simulink model "BLDC_ClosedLoop_s32k144"  (Simulink 9.0)
settings: Solver=FixedStepDiscrete  StartTime=0.0  StopTime=10.0  FixedStep=0.1  RelTol=1e-3  EnableMultiTasking=on
InitFcn:
  | mbd_s32k_consistency_checks(bdroot(gcs));
undefined symbols (not defined in the file): External, LQFP, One, Shot, TRGMUX_PDB_TRIG
libraries: mbd_s32k1xx_ec_toolbox x45, simulink x10, mbd_msd_ec_toolbox x5, ammclib_bam_s32k14x x2
(part 2 of 2)

== system BLDC_ClosedLoop_s32k144/S32K144 EVB/10us_interrupt/MeasureHallSignal_HighEdge_Time/reset counter ==
  Action Port : ActionPort  ActionPortLabel=else
  Data Store Write : DataStoreWrite  DataStoreName=SPD_COUNTS
  zero : Constant  Value=0  OutDataTypeStr=uint32
  wires:
  zero/1 -> Data Store Write/1

== system BLDC_ClosedLoop_s32k144/S32K144 EVB/Control_Logic/enable_FTM_PDB_ADC_triggering/Custom code to reload the PDB value ==

== system BLDC_ClosedLoop_s32k144/S32K144 EVB/Event_Control/ControlEventLogic/Function-Call Subsystem ==
  function : TriggerPort  TriggerType=function-call  VariantControl=Variant
  Add : Sum  AccumDataTypeStr=uint32
  Constant : Constant  OutDataTypeStr=uint32
  Data Store Read : DataStoreRead  DataStoreName=HallChangeCount  DataStoreElements=HallChangeCount
  Data Store Write : DataStoreWrite  DataStoreName=HallChangeCount  DataStoreElements=HallChangeCount
  Function-Call Generator : simulink/Ports & Subsystems/Function-Call Generator  sample_time=-1  numberOfIterations=1
  Call : Outport
  wires:
  Function-Call Generator/1 -> Call/1
  Data Store Read/1 -> Add/1
  Constant/1 -> Add/2
  Add/1 -> Data Store Write/1

== system BLDC_ClosedLoop_s32k144/S32K144 EVB/Event_Control/ControlEventLogic/Toggle_HallA ==
  function : TriggerPort  TriggerType=function-call  VariantControl=Variant
  Data Store Read1 : DataStoreRead  DataStoreName=Hall_A_sensor
  Data Store Write1 : DataStoreWrite  DataStoreName=Hall_A_sensor
  Function-Call Generator : simulink/Ports & Subsystems/Function-Call Generator  sample_time=-1  numberOfIterations=1
  Logical Operator : Logic  Operator=NOT  AllPortsSameDT=off  OutDataTypeStr=boolean
  Call : Outport
  wires:
  Function-Call Generator/1 -> Call/1
  Data Store Read1/1 -> Logical Operator/1
  Logical Operator/1 -> Data Store Write1/1

== system BLDC_ClosedLoop_s32k144/S32K144 EVB/Event_Control/ControlEventLogic/Toggle_HallB ==
  function : TriggerPort  TriggerType=function-call  VariantControl=Variant
  Data Store Read1 : DataStoreRead  DataStoreName=Hall_B_sensor
  Data Store Write1 : DataStoreWrite  DataStoreName=Hall_B_sensor
  Function-Call Generator : simulink/Ports & Subsystems/Function-Call Generator  sample_time=-1  numberOfIterations=1
  Logical Operator : Logic  Operator=NOT  AllPortsSameDT=off  OutDataTypeStr=boolean
  Call : Outport
  wires:
  Function-Call Generator/1 -> Call/1
  Data Store Read1/1 -> Logical Operator/1
  Logical Operator/1 -> Data Store Write1/1

== system BLDC_ClosedLoop_s32k144/S32K144 EVB/Event_Control/ControlEventLogic/Toggle_HallC ==
  function : TriggerPort  TriggerType=function-call  VariantControl=Variant
  Data Store Read1 : DataStoreRead  DataStoreName=Hall_C_sensor
  Data Store Write1 : DataStoreWrite  DataStoreName=Hall_C_sensor
  Function-Call Generator : simulink/Ports & Subsystems/Function-Call Generator  sample_time=-1  numberOfIterations=1
  Logical Operator : Logic  Operator=NOT  AllPortsSameDT=off  OutDataTypeStr=boolean
  Call : Outport
  wires:
  Function-Call Generator/1 -> Call/1
  Data Store Read1/1 -> Logical Operator/1
  Logical Operator/1 -> Data Store Write1/1

== system BLDC_ClosedLoop_s32k144/S32K144 EVB/Hall_Emulation_Sequence/Speed Estimator/keep updating history ==
  Action Port : ActionPort  ActionPortLabel=else
  Data Store Read : DataStoreRead  DataStoreName=Hall_A_sensor
  Data Store Write3 : DataStoreWrite  DataStoreName=HALL_A_Input_1
  wires:
  Data Store Read/1 -> Data Store Write3/1

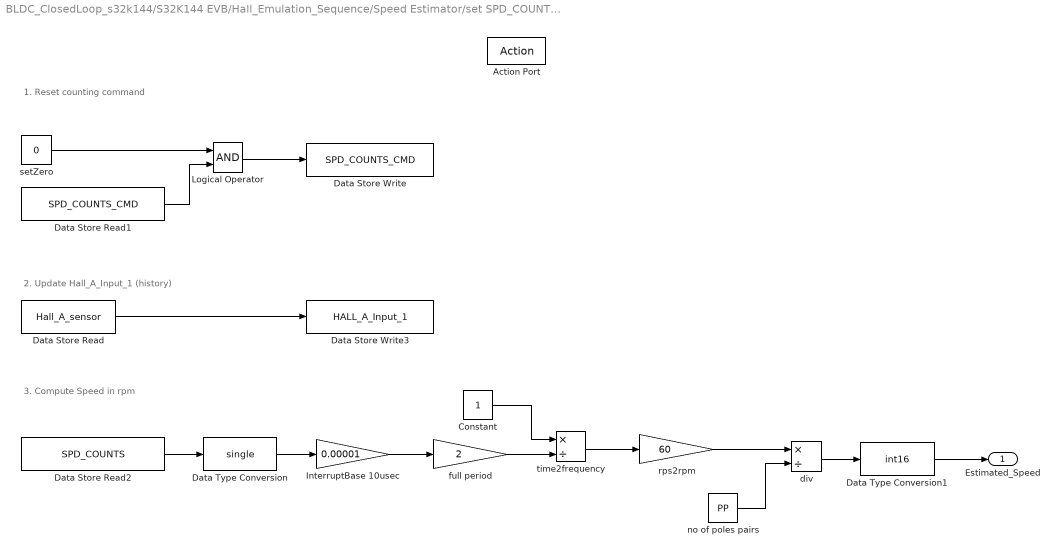
== system BLDC_ClosedLoop_s32k144/S32K144 EVB/Hall_Emulation_Sequence/Speed Estimator/set SPD_COUNT_CMD = 0 ==
  note: 2. Update Hall_A_Input_1 (history)
  note: 1. Reset counting command
  note: 3. Compute Speed in rpm
  Action Port : ActionPort  ActionPortLabel=elseif((u1 == 0)&(u2 == 1))
  Constant : Constant  OutDataTypeStr=single
  Data Store Read : DataStoreRead  DataStoreName=Hall_A_sensor
  Data Store Read1 : DataStoreRead  DataStoreName=SPD_COUNTS_CMD
  Data Store Read2 : DataStoreRead  DataStoreName=SPD_COUNTS
  Data Store Write : DataStoreWrite  DataStoreName=SPD_COUNTS_CMD
  Data Store Write3 : DataStoreWrite  DataStoreName=HALL_A_Input_1
  Data Type Conversion : DataTypeConversion  OutDataTypeStr=single
  Data Type Conversion1 : DataTypeConversion  OutDataTypeStr=int16
  InterruptBase 10usec : Gain  Gain=0.00001  OutDataTypeStr=single
  Logical Operator : Logic  AllPortsSameDT=off  OutDataTypeStr=boolean
  div : Product  Inputs=*/  OutDataTypeStr=single
  full period : Gain  Gain=2  OutDataTypeStr=single
  no of poles pairs : Constant  Value=PP  OutDataTypeStr=single
  rps2rpm : Gain  Gain=60  OutDataTypeStr=single
  setZero : Constant  Value=0  OutDataTypeStr=boolean
  time2frequency : Product  Inputs=*/  OutDataTypeStr=single
  Estimated_Speed : Outport
  wires:
  Data Store Read/1 -> Data Store Write3/1
  Logical Operator/1 -> Data Store Write/1
  setZero/1 -> Logical Operator/1
  Data Store Read1/1 -> Logical Operator/2
  Data Store Read2/1 -> Data Type Conversion/1
  Data Type Conversion/1 -> InterruptBase 10usec/1
  InterruptBase 10usec/1 -> full period/1
  full period/1 -> time2frequency/2
  Constant/1 -> time2frequency/1
  time2frequency/1 -> rps2rpm/1
  rps2rpm/1 -> div/1
  no of poles pairs/1 -> div/2
  div/1 -> Data Type Conversion1/1
  Data Type Conversion1/1 -> Estimated_Speed/1

== system BLDC_ClosedLoop_s32k144/S32K144 EVB/Hall_Emulation_Sequence/Speed Estimator/set SPD_COUNT_CMD = 1 ==
  note: 2. Update Hall_A_Input_1 (history)
  note: 1. Enable counting command
  Action Port : ActionPort  ActionPortLabel=if((u1 == 1)&(u2 == 0))
  Data Store Read : DataStoreRead  DataStoreName=Hall_A_sensor
  Data Store Read1 : DataStoreRead  DataStoreName=SPD_COUNTS_CMD
  Data Store Write : DataStoreWrite  DataStoreName=SPD_COUNTS_CMD
  Data Store Write3 : DataStoreWrite  DataStoreName=HALL_A_Input_1
  Logical Operator : Logic  Operator=OR  AllPortsSameDT=off  OutDataTypeStr=boolean
  setOne : Constant  OutDataTypeStr=boolean
  wires:
  Data Store Read/1 -> Data Store Write3/1
  Logical Operator/1 -> Data Store Write/1
  setOne/1 -> Logical Operator/1
  Data Store Read1/1 -> Logical Operator/2

== system BLDC_ClosedLoop_s32k144/S32K144 EVB/IO Controls /Subsystem/Fault ==
  Action Port : ActionPort  ActionPortLabel=elseif((u2 == 1))
  BLUE : mbd_s32k1xx_ec_toolbox/GPIO Blocks/Digital_Output  gpio_pin=PTD0: [PTD0 | Port D I/O]  init_val=Low  drive_strength=Low
  GREEN : mbd_s32k1xx_ec_toolbox/GPIO Blocks/Digital_Output  gpio_pin=PTD16: [PTD16 | Port D I/O]  init_val=Low  drive_strength=Low
  OFF : Constant  OutDataTypeStr=boolean
  "OFF " : Constant  OutDataTypeStr=boolean
  "OFF  " : Constant  Value=0  OutDataTypeStr=boolean
  "ON " : Constant  Value=0  OutDataTypeStr=boolean
  RED : mbd_s32k1xx_ec_toolbox/GPIO Blocks/Digital_Output  gpio_pin=PTD15: [PTD15 | Port D I/O]  init_val=Low  drive_strength=Low
  "SpeedCmd " : DataStoreWrite  DataStoreName=START
  SpeedCmd 1 : DataStoreWrite  DataStoreName=READY
  wires:
  "OFF "/1 -> GREEN/1
  "ON "/1 -> RED/1
  OFF/1 -> BLUE/1
  "OFF  "/1 -> "SpeedCmd "/1, SpeedCmd 1/1

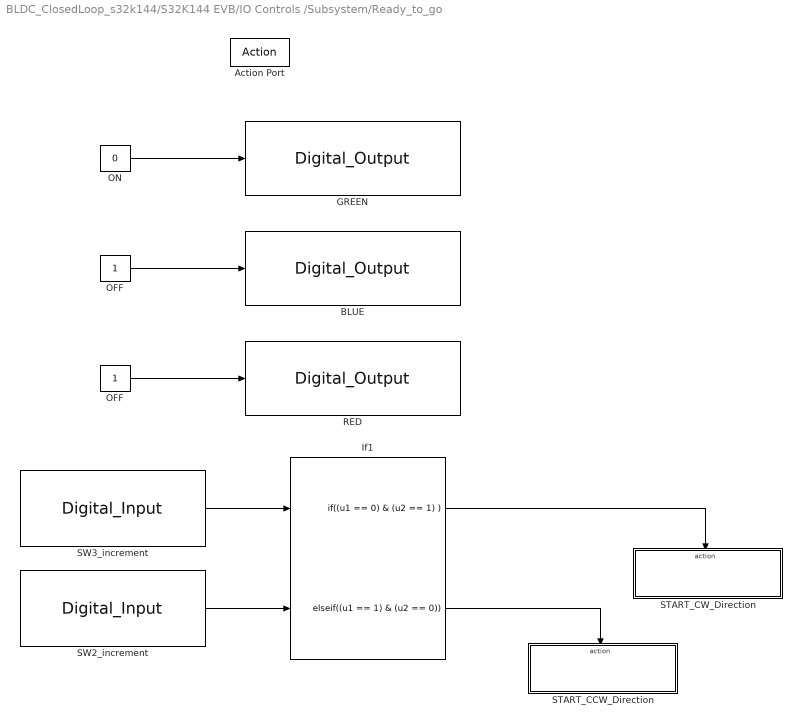
== system BLDC_ClosedLoop_s32k144/S32K144 EVB/IO Controls /Subsystem/Ready_to_go ==
  Action Port : ActionPort  ActionPortLabel=if((u1 == 0) & (u2 == 0))
  BLUE : mbd_s32k1xx_ec_toolbox/GPIO Blocks/Digital_Output  gpio_pin=PTD0: [PTD0 | Port D I/O]  init_val=Low  drive_strength=Low
  GREEN : mbd_s32k1xx_ec_toolbox/GPIO Blocks/Digital_Output  gpio_pin=PTD16: [PTD16 | Port D I/O]  init_val=Low  drive_strength=Low
  If1 : If  NumInputs=2  IfExpression=(u1 == 0) & (u2 == 1)  ElseIfExpressions=(u1 == 1) & (u2 == 0)  ShowElse=off
  "OFF " : Constant  OutDataTypeStr=boolean
  "OFF  " : Constant  OutDataTypeStr=boolean
  "ON  " : Constant  Value=0  OutDataTypeStr=boolean
  RED : mbd_s32k1xx_ec_toolbox/GPIO Blocks/Digital_Output  gpio_pin=PTD15: [PTD15 | Port D I/O]  init_val=Low  drive_strength=Low
  START_CCW_Direction : Subsystem  TreatAsAtomicUnit=on
  START_CW_Direction : Subsystem  TreatAsAtomicUnit=on
  SW2_increment : mbd_s32k1xx_ec_toolbox/GPIO Blocks/Digital_Input  gpio_pin=PTC12: [PTC12 | Port C I/O]  pull_resistor=None  passive_filter=off
  SW3_increment : mbd_s32k1xx_ec_toolbox/GPIO Blocks/Digital_Input  gpio_pin=PTC13: [PTC13 | Port C I/O]  pull_resistor=None  passive_filter=off
  wires:
  "ON  "/1 -> GREEN/1
  "OFF "/1 -> RED/1
  "OFF  "/1 -> BLUE/1
  If1/1 -> START_CW_Direction/Action
  SW3_increment/1 -> If1/1
  SW2_increment/1 -> If1/2
  If1/2 -> START_CCW_Direction/Action

== system BLDC_ClosedLoop_s32k144/S32K144 EVB/IO Controls /Subsystem/Running ==
  Action Port : ActionPort  ActionPortLabel=else
  BLUE : mbd_s32k1xx_ec_toolbox/GPIO Blocks/Digital_Output  gpio_pin=PTD0: [PTD0 | Port D I/O]  init_val=Low  drive_strength=Low
  GREEN : mbd_s32k1xx_ec_toolbox/GPIO Blocks/Digital_Output  gpio_pin=PTD16: [PTD16 | Port D I/O]  init_val=Low  drive_strength=Low
  "OFF " : Constant  OutDataTypeStr=boolean
  OFF_RED : Constant  OutDataTypeStr=boolean
  "ON " : Constant  Value=0  OutDataTypeStr=boolean
  RED : mbd_s32k1xx_ec_toolbox/GPIO Blocks/Digital_Output  gpio_pin=PTD15: [PTD15 | Port D I/O]  init_val=Low  drive_strength=Low
  wires:
  "OFF "/1 -> GREEN/1
  OFF_RED/1 -> RED/1
  "ON "/1 -> BLUE/1

== system BLDC_ClosedLoop_s32k144/S32K144 EVB/Protection_Check/Subsystem/FAILURE ==
  Action Port : ActionPort  ActionPortLabel=if((u1 < VDC_UNDERVOLTAGE) | (u1 > VDC_OVERVOLTAGE) | (u2 > IDC_OVERCURRENT))
  FAULT_write : DataStoreWrite  DataStoreName=FAULT
  FTM_PWM_Disable_Enable : mbd_s32k1xx_ec_toolbox/Motor Control Blocks/FTM Blocks/FTM_PWM_Disable_Enable  ftmModule=3  action=Disable
  NOK : Constant  OutDataTypeStr=boolean
  TPP_Functional_Mode : mbd_msd_ec_toolbox/TPP/TPP_Functional_Mode  tppInstance=0  action=Sleep
  wires:
  NOK/1 -> FAULT_write/1

== system BLDC_ClosedLoop_s32k144/S32K144 EVB/Trapezoidal_Control/SixStepCommutationLogic/Alignment_Counter ==
  Action Port : ActionPort  ActionPortLabel=if((u1 == 1))
  Align Sequence : Stateflow chart  TreatAsAtomicUnit=on
  AlignTimerIn : DataStoreRead  DataStoreName=AlignTimer
  AlignTimerOut : DataStoreWrite  DataStoreName=AlignTimer
  ExecureAlign : DataStoreWrite  DataStoreName=ExecuteAlign
  wires:
  Align Sequence/2(ExecuteAlign) -> ExecureAlign/1
  Align Sequence/1(DelayTimeOut) -> AlignTimerOut/1
  AlignTimerIn/1 -> Align Sequence/1(DelayTimeIn)

== system BLDC_ClosedLoop_s32k144/S32K144 EVB/Trapezoidal_Control/SixStepCommutationLogic/Do_Alignment ==
  DIR : Inport
  Action Port : ActionPort  ActionPortLabel=if((u1 == 1) & (u2 == 0) & (u3 == 1))
  CCW Dir : Subsystem
  CW Dir : Subsystem
  DirectionChk : If  Priority=1  IfExpression=(u1 >= 0)
  Merge : Merge
  Merge1 : Merge
  Merge2 : Merge
  Phase_A : Outport
  Phase_B : Outport  Port=2
  Phase_C : Outport  Port=3
  wires:
  DIR/1 -> DirectionChk/1
  DirectionChk/1 -> CW Dir/Action
  DirectionChk/2 -> CCW Dir/Action
  Merge/1 -> Phase_A/1
  Merge1/1 -> Phase_C/1
  CCW Dir/3(Out3) -> Merge1/2
  CW Dir/3(Out3) -> Merge1/1
  CW Dir/1(Out1) -> Merge/1
  CCW Dir/1(Out1) -> Merge/2
  CW Dir/2(Out2) -> Merge2/1
  CCW Dir/2(Out2) -> Merge2/2
  Merge2/1 -> Phase_B/1

== system BLDC_ClosedLoop_s32k144/S32K144 EVB/Trapezoidal_Control/SixStepCommutationLogic/Normal_Run ==
  DIR : Inport
  HALL_STATE : Inport  Port=2
  Action Port : ActionPort  ActionPortLabel=elseif((u1 == 0) & (u2 > 0) & (u3 == 1))
  CommutationTableLookup : Stateflow chart  TreatAsAtomicUnit=on
  Phase_A : Outport
  Phase_B : Outport  Port=2
  Phase_C : Outport  Port=3
  wires:
  CommutationTableLookup/2(Phase_B) -> Phase_B/1
  DIR/1 -> CommutationTableLookup/2(DIR)
  HALL_STATE/1 -> CommutationTableLookup/1(HALL_STATE)
  CommutationTableLookup/3(Phase_C) -> Phase_C/1
  CommutationTableLookup/1(Phase_A) -> Phase_A/1

== system BLDC_ClosedLoop_s32k144/S32K144 EVB/IO Controls /Subsystem/Ready_to_go/START_CCW_Direction ==
  Action Port : ActionPort  ActionPortLabel=elseif((u1 == 1) & (u2 == 0) )
  Constant : Constant  Value=-S0  OutDataTypeStr=Inherit: Inherit via back propagation
  ON : Constant  OutDataTypeStr=boolean
  PIT_Counter_Start_Stop : mbd_s32k1xx_ec_toolbox/Utility Blocks/PIT_Counter_Start_Stop  channel=1  action=Start
  PIT_Interrupt_Enable_Disable : mbd_s32k1xx_ec_toolbox/Utility Blocks/PIT_Interrupt_Enable_Disable  channel=1  enable=on
  "SpeedCmd " : DataStoreWrite  DataStoreName=START
  Store Command : DataStoreWrite  DataStoreName=SpeedReqCMD
  wires:
  Constant/1 -> Store Command/1
  ON/1 -> "SpeedCmd "/1

== system BLDC_ClosedLoop_s32k144/S32K144 EVB/IO Controls /Subsystem/Ready_to_go/START_CW_Direction ==
  Action Port : ActionPort  ActionPortLabel=if((u1 == 0) & (u2 == 1) )
  Constant : Constant  Value=S0  OutDataTypeStr=Inherit: Inherit via back propagation
  ON : Constant  OutDataTypeStr=boolean
  PIT_Counter_Start_Stop : mbd_s32k1xx_ec_toolbox/Utility Blocks/PIT_Counter_Start_Stop  channel=1  action=Start
  PIT_Interrupt_Enable_Disable : mbd_s32k1xx_ec_toolbox/Utility Blocks/PIT_Interrupt_Enable_Disable  channel=1  enable=on
  "SpeedCmd " : DataStoreWrite  DataStoreName=START
  Store Command : DataStoreWrite  DataStoreName=SpeedReqCMD
  wires:
  ON/1 -> "SpeedCmd "/1
  Constant/1 -> Store Command/1

== system BLDC_ClosedLoop_s32k144/S32K144 EVB/Trapezoidal_Control/SixStepCommutationLogic/Do_Alignment/CCW Dir ==
  Action Port : ActionPort  ActionPortLabel=else
  Constant : Constant  OutDataTypeStr=Inherit: Inherit via back propagation
  Constant1 : Constant  Value=0  OutDataTypeStr=Inherit: Inherit via back propagation
  Constant2 : Constant  Value=2  OutDataTypeStr=Inherit: Inherit via back propagation
  Out1 : Outport
  Out2 : Outport  Port=2
  Out3 : Outport  Port=3
  wires:
  Constant1/1 -> Out2/1
  Constant2/1 -> Out3/1
  Constant/1 -> Out1/1

== system BLDC_ClosedLoop_s32k144/S32K144 EVB/Trapezoidal_Control/SixStepCommutationLogic/Do_Alignment/CW Dir ==
  Action Port : ActionPort  ActionPortLabel=if((u1 >= 0))
  Constant : Constant  Value=2  OutDataTypeStr=Inherit: Inherit via back propagation
  Constant1 : Constant  Value=0  OutDataTypeStr=Inherit: Inherit via back propagation
  Constant2 : Constant  OutDataTypeStr=Inherit: Inherit via back propagation
  Out1 : Outport
  Out2 : Outport  Port=2
  Out3 : Outport  Port=3
  wires:
  Constant/1 -> Out1/1
  Constant2/1 -> Out3/1
  Constant1/1 -> Out2/1

== stateflow chart S32K144 EVB/Trapezoidal_Control/SixStepCommutationLogic/Alignment_Counter/Align Sequence ==
  settings: sampleTime=0.500
  (default) -> (junction 7)
  (junction 7) -> (junction 8) [order 1] : [DelayTimeIn > ALIGN_TIME]
      | {ExecuteAlign = 0;}
  (junction 7) -> (junction 9) [order 2]
  (junction 8) -> (junction 10)
  (junction 9) -> (junction 10) : {DelayTimeOut = DelayTimeIn + 1;
      | ExecuteAlign = 1;}
  data: DelayTimeOut output uint16; DelayTimeIn input uint16; ExecuteAlign output boolean; ALIGN_TIME parameter double

== stateflow chart S32K144 EVB/Control_Logic/Enable PDB and start FTM ==
  settings: sampleTime=0.500
  state END
  state A
  (default) -> A
  A -> END : /*Post initializations*/
      | {enablePDB;}
  END -> END : {Normal_Op;}
  events: enablePDB output FUNCTION_CALL_EVENT; Normal_Op output FUNCTION_CALL_EVENT

== stateflow chart S32K144 EVB/Event_Control/ControlPollingLogic ==
  state Logic1
    Logic1 -> (junction 28)
    (default) -> (junction 28)
    (junction 28) -> (junction 29) [order 1] : [(SpeedChange <= S0) && (SpeedChange >= -S0)]
        | {Trigger;}
    (junction 28) -> (junction 30) [order 2]
    (junction 29) -> (junction 31)
    (junction 30) -> (junction 31)
  (default) -> Logic1
  data: SpeedChange input int16; S0 parameter double
  events: Trigger output FUNCTION_CALL_EVENT

== stateflow chart S32K144 EVB/IO Controls /If Action Subsystem/Chart ==
  state SwitchCheck1 [parallel]
    settings: executionOrder=1
    state Decrement
      du:out = 0;
      (default) -> (junction 50)
      Decrement -> (junction 50) [order 1] : [((Increment ==0)& ...
          |  (Decrement==1))& hasChanged(Increment)]
          | {out=-100;}
    state Increment
      du:out = 0;
      (default) -> (junction 53)
      Increment -> (junction 53) [order 1] : [((Increment ==1)& ...
          |  (Decrement==0))&hasChanged(Decrement)]
          | {out=100;}
    (default) -> Decrement : { out =0;}
    Increment -> Decrement [order 1] : [(Increment==0)& ...
        |  (Decrement==1) ...
        | & hasChanged(Increment)]
        | {out=-100;}
    Decrement -> Increment [order 1] : [((Increment ==1)& ...
        |  (Decrement==0))&hasChanged(Decrement)]
        | {out=100;}
  data: out output int16; Increment input boolean; Decrement input boolean

== stateflow chart S32K144 EVB/Trapezoidal_Control/SixStepCommutationLogic/Normal_Run/CommutationTableLookup ==
  (default) -> (junction 68)
  (junction 68) -> (junction 69) [order 1] : /*CCW*/
      | [DIR < 0]
  (junction 68) -> (junction 70) [order 2] : /*CW*/
      | [DIR >= 0]
  (junction 69) -> (junction 71) : {
      |    Phase_A = ccwTable[HALL_STATE][0];
      |    Phase_B = ccwTable[HALL_STATE][1];
      |    Phase_C = ccwTable[HALL_STATE][2];
      | }
  (junction 70) -> (junction 71) : {
      |    Phase_A = cwTable[HALL_STATE][0];
      |    Phase_B = cwTable[HALL_STATE][1];
      |    Phase_C = cwTable[HALL_STATE][2];
      | }
  data: ccwTable constant uint8 size=[8 3] =[0 0 0; 0 2 1; 2 1 0; 2 0 1; 1 0 2; 1 2 0; 0 1 2; 0 0 0;]; HALL_STATE input uint8; Phase_A output uint8; Phase_B output uint8; Phase_C output uint8; cwTable constant uint8 size=[8 3] =[0 0 0; 0 1 2; 1 2 0; 1 0 2; 2 0 1; 2 1 0; 0 2 1; 0 0 0;]; DIR input int16

== stateflow chart S32K144 EVB/Trapezoidal_Control/PhaseSwitchLogic ==
  settings: sampleTime=0.500
  note: Phase States:
      | 0 = NC
      | 1 = -Vdcb
      | 2 = +Vdcb
  (default) -> (junction 90)
  (junction 90) -> (junction 91) [order 1] : /*check for phase state 0 */
      | [Phase_A == 0]
      | /*set output for state 0 */
      | {Phase_A_HS = 0; Phase_A_LS =0;}
  (junction 90) -> (junction 92) [order 2]
  (junction 91) -> (junction 93)
  (junction 92) -> (junction 93) [order 1] : /*check for phase state 1 */
      | [Phase_A == 1]
      | /*set output for state 1 */
      | {Phase_A_HS = 0; Phase_A_LS = PWM_Duty_Cycle;}
  (junction 92) -> (junction 94) [order 2]
  (junction 93) -> (junction 95)
  (junction 94) -> (junction 95) [order 1] : /*check for phase state 2 */
      | [Phase_A == 2]
      | /*set output for state 2 */
      | {Phase_A_HS = 1; Phase_A_LS = 0;}
  (junction 94) -> (junction 96) [order 2]
  (junction 95) -> (junction 97)
  (junction 96) -> (junction 97)
  (junction 97) -> (junction 98) [order 1] : /*check for phase state 0 */
      | [Phase_B == 0]
      | /*set output for state 0 */
      | {Phase_B_HS = 0; Phase_B_LS = 0;}
  (junction 97) -> (junction 99) [order 2]
  (junction 98) -> (junction 100)
  (junction 99) -> (junction 100) [order 1] : /*check for phase state 1 */
      | [Phase_B == 1]
      | /*set output for state 1 */
      | {Phase_B_HS = 0; Phase_B_LS = PWM_Duty_Cycle;}
  (junction 99) -> (junction 101) [order 2]
  (junction 100) -> (junction 102)
  (junction 101) -> (junction 102) [order 1] : /*check for phase state 2 */
      | [Phase_B == 2]
      | /*set output for state 2 */
      | {Phase_B_HS = 1; Phase_B_LS = 0;}
  (junction 101) -> (junction 103) [order 2]
  (junction 102) -> (junction 104)
  (junction 103) -> (junction 104)
  (junction 104) -> (junction 105) [order 1] : /*check for phase state 0 */
      | [Phase_C == 0]
      | /*set output for state 0 */
      | {Phase_C_HS = 0; Phase_C_LS = 0;}
  (junction 104) -> (junction 106) [order 2]
  (junction 105) -> (junction 107)
  (junction 106) -> (junction 107) [order 1] : /*check for phase state 1 */
      | [Phase_C == 1]
      | /*set output for state 1 */
      | {Phase_C_HS = 0; Phase_C_LS = PWM_Duty_Cycle;}
  (junction 106) -> (junction 108) [order 2]
  (junction 107) -> (junction 109)
  (junction 108) -> (junction 109) [order 1] : /*check for phase state 2 */
      | [Phase_C == 2]
      | /*set output for state 2 */
      | {Phase_C_HS = 1; Phase_C_LS = 0;}
  (junction 108) -> (junction 110) [order 2]
  (junction 109) -> (junction 111)
  (junction 110) -> (junction 111)
  data: Phase_A input double; Phase_B input double; Phase_C input double; Phase_A_HS output single; Phase_A_LS output single; Phase_B_HS output single; Phase_B_LS output single; Phase_C_HS output single; Phase_C_LS output single; PWM_Duty_Cycle input single

== stateflow chart S32K144 EVB/Event_Control/Init ==
  settings: sampleTime=0.500
  state A
  state B
  (default) -> A
  A -> B : {Init;
      | index=0;}
  data: index local double
  events: Init output FUNCTION_CALL_EVENT

== stateflow chart S32K144 EVB/Speed_Controller/Motor_Speed_Sign/RPM_ZeroDetect ==
  state Loop_Counter
    Loop_Counter -> (junction 155)
    (default) -> (junction 155)
    (junction 155) -> (junction 154) [order 3]
    (junction 155) -> (junction 156) [order 2] : [Loop_Count >= TimeDelay]
        | {Loop_Count = 0;}
    (junction 156) -> (junction 157) [order 1] : [(HallStateChangeCount >= EdgeDetectMin)]
        | {Enable = 1;
        | ClearCount = 0;}
    (junction 156) -> (junction 160) [order 3]
    (junction 154) -> (junction 158)
    (junction 155) -> (junction 159) [order 1] : [(HallStateChangeCount >= EdgeDetectMin) && (Enable == 0)]
        | {Enable = 1;}
    (junction 156) -> (junction 160) [order 2] : [(Enable == 1)]
        | {Enable = 0;
        | ClearCount = 0;}
    (junction 157) -> (junction 161)
    (junction 158) -> (junction 159)
    (junction 159) -> (junction 160) : {ClearCount = HallStateChangeCount;}
    (junction 160) -> (junction 161) : {Loop_Count++;}
  (default) -> Loop_Counter : {Loop_Count = 0;}
  data: Loop_Count local double; TimeDelay input int16; HallStateChangeCount input uint32; EdgeDetectMin input int16; Enable output boolean; ClearCount output uint32
